simulink model "CSI_0313_SDC"  (R2019b)
settings: Solver=FixedStepDiscrete  StartTime=0.0  StopTime=Tstop  FixedStep=Tdelt  MaxStep=1e-4  RelTol=1e-3
values from neighbouring files (symbols this model uses):
  C = 12e-6    (= 1.2e-05)    [Inputparameter.m]
  Cdc = 4.76*10^-3    (= 0.00476)    [Inputparameter.m]
  Cemc = 1.5e-6    (= 1.5e-06)    [Inputparameter.m]
  enb = 0    [Run.m]
  fanalog = 7000    [Run.m]
  fTs = Update/18000    (= 0.000111111111111)    [Run.m]
  Ibase = 43*sqrt(2)    [Inputparameter.m]
  K120 = 0.0    (= 0)    [Run.m]
  K21 = 0.0    (= 0)    [Run.m]
  K5 = 0.0    (= 0)    [Run.m]
  K7 = 0.0    (= 0)    [Run.m]
  Kipll = 1.0    (= 1)    [Run.m]
  Klim = 1.03    [Run.m]
  Kpll = 20.0    (= 20)    [Run.m]
  Kpr = 0.9*Ibase/(Vbase)    [Run.m]
  Lgrid = 7.717e-4*10    (= 0.007717)    [Run.m]
  Lline = 60e-6    (= 6e-05)    [Inputparameter.m]
  Lpwm = 184.8e-6    (= 0.0001848)    [Inputparameter.m]
  mode = 1    [Run.m]
  Nsw = 18000/fbase    [Run.m]
  Qbpf = 1.0    (= 1)    [Run.m]
  Qpr = 1.0    (= 1)    [Run.m]
  Qs = 1    [Run.m]
  Rc = 10e-3    (= 0.01)    [Inputparameter.m]
  Remc = 1e-3    (= 0.001)    [Inputparameter.m]
  Rgrid = 2*pi*fbase*Lgrid/XR    [Run.m]
  Rline = 4.95e-3    (= 0.00495)    [Inputparameter.m]
  Rpre = 2.2    [Inputparameter.m]
  Rpwm = 6.2e-3    (= 0.0062)    [Inputparameter.m]
  Tdelt = (fTs)/(200*Update)    (= 2.77777777778e-07)    [Run.m]
  Tdt = 1.27e-6    (= 1.27e-06)    [Run.m]
  tstart = 0.2    [Run.m]
  Update = 2    [Run.m]
  Vbase = 400*sqrt(2/3)    [Inputparameter.m]
undefined symbols (not defined in the file or in its folder): sigbuilder_block
libraries: powerlib x54
(part 1 of 4)
settings Model: SimulationMode=accelerator  Creator=seyuoka  LastModifiedBy=INANPAN1
settings DataIOCC: ReturnWorkspaceOutputs=off
settings OptimizationCC: EfficientMapNaN2IntZero=off
settings DebuggingCC: ArithmeticOperatorsInVariantConditions=warning
settings HardwareCC: TargetBitPerPointer=64  TargetBitPerSizeT=64  TargetBitPerPtrDiffT=64  TargetLongLongMode=on  TargetIntDivRoundTo=Zero  TargetEndianess=LittleEndian  TargetWordSize=64  TargetHWDeviceType=MATLAB Host  ProdEqTarget=off
settings SFSimCC: SimUseLocalCustomCode=off  CustomCodeUndefinedFunction=UseInterfaceOnly
settings RTWCC: RTWUseLocalCustomCode=off
settings CodeAppCC: MaxIdLength=128
settings GRTTargetCC: TargetLangStandard=C89/C90 (ANSI)  CombineOutputUpdateFcns=off  GRTInterface=on
settings SimscapeCC: SimscapeNormalizeSystem=off

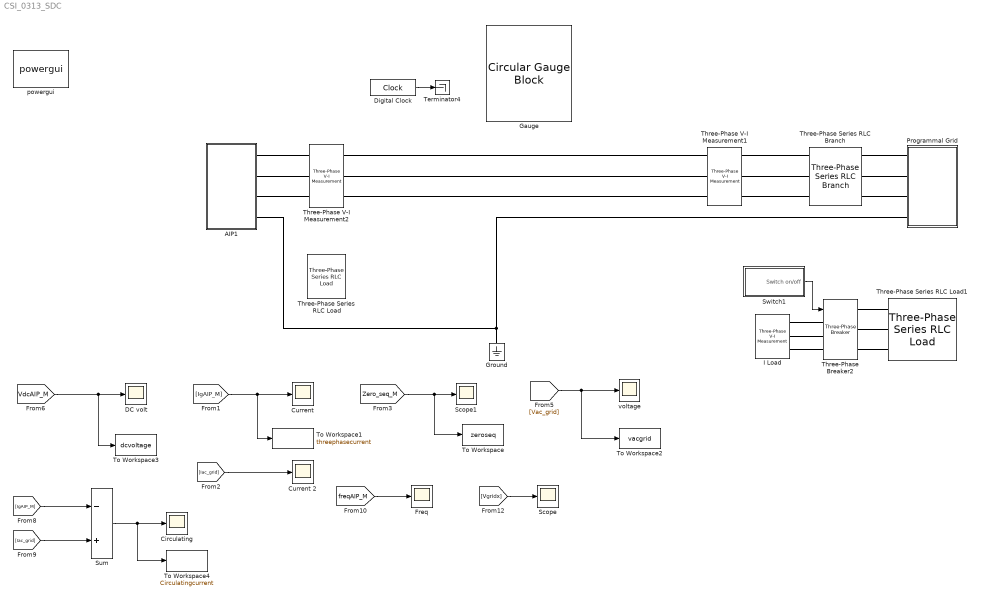
== system CSI_0313_SDC ==
  AIP1 : Subsystem
  Circulating : Scope
  "Current " : Scope
  Current 2 : Scope
  DC volt : Scope
  Digital Clock : DigitalClock  SampleTime=0.001
  Freq : Scope
  Gauge : CircularGaugeBlock  ScaleMax=1  TickInterval=0.1
  Ground : powerlib/Elements/Ground  LConnTagsString=a
      settings: SourceProductName=Simscape Electrical
  I Load : powerlib/Measurements/Three-Phase V-I Measurement  VoltageMeasurement=phase-to-ground  SetLabelV=on  LabelV=VLoad  Vpu=off  VpuLL=off  CurrentMeasurement=yes  SetLabelI=on  LabelI=ILoad  Ipu=off  Pbase=100e6  Vbase=500e3  OutputType=Complex  PhasorSimulation=off  PSBequivalent=0
      settings: SourceProductName=Simscape Electrical
  Programmal Grid : Subsystem  AncestorBlock=AIP_Library0107/Programmal Grid
  Scope : Scope
  Scope1 : Scope
  Sum : Sum  Inputs=-+
  Switch1 : Subsystem  Tag=STV Subsys  LoadFcn=sigbuilder_block('load');  StartFcn=sigbuilder_block('start');  StopFcn=sigbuilder_block('stop');  ClipboardFcn=sigbuilder_block('clipboard');  mask(Sigbuilder block){tuvar=[0:10]}
      mask help: Simulink:masks:SigbuilderBlock_MD
      mask init:
      | if ~strcmp(get_param(bdroot(gcbh),'SimulationStatus'),'stopped') tuvar = sigbuilder_block('maskInit'); end
      settings: CopyFcn=sigbuilder_block('copy');  DeleteFcn=sigbuilder_block('delete');  ModelCloseFcn=sigbuilder_block('modelClose');  PreSaveFcn=sigbuilder_block('preSave');  PauseFcn=sigbuilder_block('pause');  ContinueFcn=sigbuilder_block('continue');  NameChangeFcn=sigbuilder_block('namechange');  OpenFcn=sigbuilder_block('open',[467 144 551 302 ]);  CloseFcn=sigbuilder_block('close');
      mask Display: plot(0, 0, 100, 100,[2, 2, 32, 32, 2], [68, 8, 8, 68, 68],[32, 2], [38, 38], [32, 19, 2],[53, 60, 44], [32, 17, 17, 2],[16, 16, 31, 31]);txt = getActiveGroup(gcbh);text(2, 100, txt,'verticalAlignment', 'top');
  Terminator4 : Terminator
  Three-Phase Series RLC Branch : powerlib/Elements/Three-Phase Series RLC Branch  LConnTagsString=A|B|C  RConnTagsString=A|B|C  BranchType=RL  Resistance=Rgrid  Inductance=Lgrid  Capacitance=1e-6  Measurements=None
      settings: SourceProductName=Simscape Electrical
  Three-Phase Series RLC Load : powerlib/Elements/Three-Phase Series RLC Load  LConnTagsString=A|B|C  Configuration=Y (floating)  NominalVoltage=400  Vabc=[1e3 1e3 1e3]  Vabcp=[1e3 1e3 1e3]  NominalFrequency=50  UnbalancedPower=off  ActivePower=5000  InductivePower=0  CapacitivePower=0  Pabc=[10e3 9e3 11e3]  QLabc=[100 90 110]  QCabc=[100 90 110]  Pabcp=[10e3 9e3 11e3]  QLabcp=[100 90 110]  QCabcp=[100 90 110]  Measurements=None  LoadType=constant Z
      settings: SourceProductName=Simscape Electrical
  Three-Phase Series RLC Load1 : powerlib/Elements/Three-Phase Series RLC Load  LConnTagsString=A|B|C  Configuration=Y (grounded)  NominalVoltage=400  Vabc=[230 230 230]  Vabcp=[400 400 400]  NominalFrequency=50  UnbalancedPower=off  ActivePower=6e3  InductivePower=20e3  CapacitivePower=0  Pabc=[1 3e3 1]  QLabc=[0 16e3 0]  QCabc=[0 0 0]  Pabcp=[1 3e3 1]  QLabcp=[0 6e3 0]  QCabcp=[0 0 0]  Measurements=None  LoadType=constant Z
      settings: SourceProductName=Simscape Electrical
  Three-Phase V-I Measurement1 : powerlib/Measurements/Three-Phase V-I Measurement  VoltageMeasurement=phase-to-ground  SetLabelV=on  LabelV=Vac_grid  Vpu=off  VpuLL=off  CurrentMeasurement=yes  SetLabelI=on  LabelI=Iac_grid  Ipu=off  Pbase=100e6  Vbase=500e3  OutputType=Complex  PhasorSimulation=off  PSBequivalent=0
      settings: SourceProductName=Simscape Electrical
  Three-Phase V-I Measurement2 : powerlib/Measurements/Three-Phase V-I Measurement  VoltageMeasurement=no  SetLabelV=on  LabelV=vacgrid  Vpu=off  VpuLL=off  CurrentMeasurement=yes  SetLabelI=on  LabelI=IgAIP_M  Ipu=off  Pbase=100e6  Vbase=500e3  OutputType=Complex  PhasorSimulation=off  PSBequivalent=0
      settings: SourceProductName=Simscape Electrical
  Three-Phase Breaker2 : powerlib/Elements/Three-Phase Breaker  InitialState=open  SwitchA=on  SwitchB=on  SwitchC=on  SwitchTimes=1.2  External=on  BreakerResistance=0.01  SnubberResistance=1e6  SnubberCapacitance=inf  Measurements=None
      settings: SourceProductName=Simscape Electrical
  To Workspace : ToWorkspace  VariableName=zeroseq  SaveFormat=Timeseries  SampleTime=-1
  To Workspace1 : ToWorkspace  VariableName=threephasecurrent  SaveFormat=Timeseries  SampleTime=-1
  To Workspace2 : ToWorkspace  VariableName=vacgrid  SaveFormat=Timeseries  SampleTime=-1
  To Workspace3 : ToWorkspace  VariableName=dcvoltage  SaveFormat=Timeseries  SampleTime=-1
  To Workspace4 : ToWorkspace  VariableName=Circulatingcurrent  SaveFormat=Timeseries  SampleTime=-1
  powergui : powerlib/powergui  Priority=1  SimulationMode=Discrete  SampleTime=Tdelt  frequency=50  Iterations=50  frequencyindice=0  Pbase=100e6  ErrMax=1e-4  UnitsV=kV  UnitsW=MW  buscounter=0  FunctionMessages=off  echomessages=off  EnableUseOfTLC=off  CurrentSourceSwitches=off  DisableSnubberDevices=off  DisableRonSwitches=off  DisableVfSwitches=off  DisplayEquations=off  AutomaticDiscreteSolvers=off  SolverType=Tustin/Backward Euler (TBE)  Interpol=off  ExternalGateDelay=off  methode=off  Ts=100  x0status=blocks  SPID=off  SwTol=0  HookPort=off  NonlinearTolerance=1e-4  nMaxIteration=100  ContinueOnMaxIteration=off  RestoreLinks=warning  ResistiveCurrentMeasurement=off  Frange=[0:2:500]  Ylog=off  Xlog=on  ShowGrid=off  save=off  variable=ZData  structure=AIPcurrent  ZoomFFT=on  StartTime=0.8  cycles=5  DisplayStyle=1  fundamental=50  FreqAxis=off  MaxFrequency=5000  frequencyindicesteady=1  RmsSteady=1  display=off
      settings: SourceProductName=Simscape Electrical
  voltage : Scope
  wires:
  Digital Clock/1 -> Terminator4/1
  [Vac_grid] -> voltage/1, To Workspace2/1
  [IgAIP_M] -> Sum/1
  [Iac_grid] -> Sum/2
  Sum/1 -> To Workspace4/1, Circulating/1
  [freqAIP_M] -> Freq/1
  [Vgridx] -> Scope/1
  [VdcAIP_M] -> To Workspace3/1, DC volt/1
  [IgAIP_M] -> To Workspace1/1, "Current "/1
  [Zero_seq_M] -> Scope1/1, To Workspace/1
  [Iac_grid] -> Current 2/1
  Switch1/1(Switch on/off) -> Three-Phase Breaker2/1
  connections:
  Three-Phase V-I Measurement2/RConn1 -- Three-Phase V-I Measurement1/LConn1
  Three-Phase V-I Measurement1/LConn3 -- Three-Phase V-I Measurement2/RConn3
  Three-Phase V-I Measurement2/RConn2 -- Three-Phase V-I Measurement1/LConn2
  Three-Phase V-I Measurement1/RConn1 -- Three-Phase Series RLC Branch/LConn1
  Three-Phase V-I Measurement1/RConn2 -- Three-Phase Series RLC Branch/LConn2
  Three-Phase V-I Measurement1/RConn3 -- Three-Phase Series RLC Branch/LConn3
  Programmal Grid/RConn4 -- AIP1/RConn4 -- Ground/LConn1
  Three-Phase Series RLC Branch/RConn3 -- Programmal Grid/RConn3
  Three-Phase Series RLC Branch/RConn2 -- Programmal Grid/RConn2
  Three-Phase Series RLC Branch/RConn1 -- Programmal Grid/RConn1
  Three-Phase V-I Measurement2/LConn1 -- AIP1/RConn1
  Three-Phase V-I Measurement2/LConn2 -- AIP1/RConn2
  Three-Phase V-I Measurement2/LConn3 -- AIP1/RConn3
  Three-Phase Series RLC Load1/LConn3 -- Three-Phase Breaker2/RConn3
  I Load/RConn1 -- Three-Phase Breaker2/LConn1
  I Load/RConn2 -- Three-Phase Breaker2/LConn2
  Three-Phase Series RLC Load1/LConn2 -- Three-Phase Breaker2/RConn2
  I Load/RConn3 -- Three-Phase Breaker2/LConn3
  Three-Phase Series RLC Load1/LConn1 -- Three-Phase Breaker2/RConn1

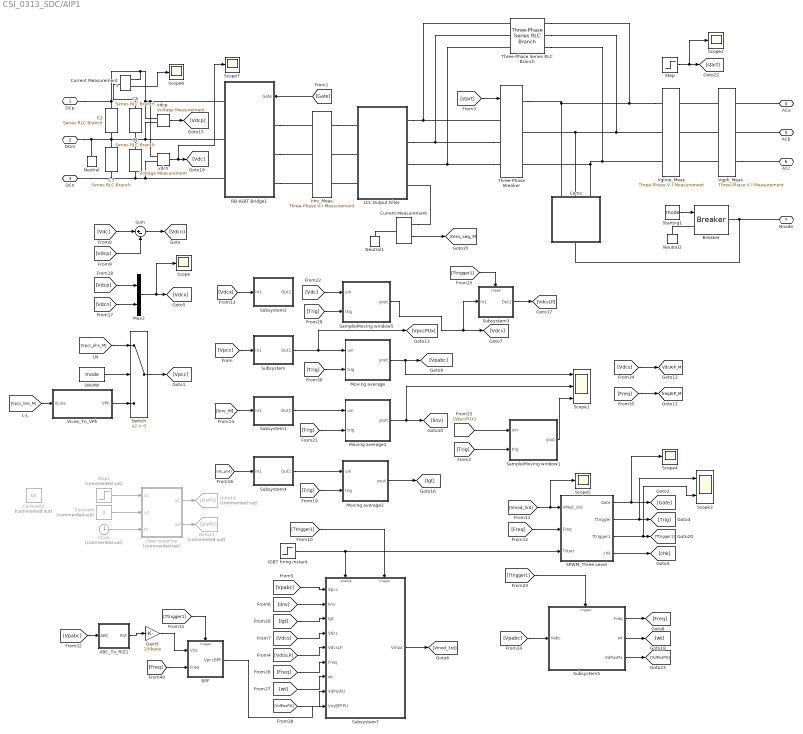
== system CSI_0313_SDC/AIP1 ==
  3W/4W : Constant  Value=mode
  ABC_To_RIZ1 : MATLAB Function  TreatAsAtomicUnit=on
  "BPF " : Subsystem
  Breaker : powerlib/Elements/Breaker  InitialState=0  SwitchingTimes="[1/60  5/60]"  External=on  BreakerResistance=1e-6  SnubberResistance=1e6  SnubberCapacitance=inf  Measurements=None  MoreParameters=on  NoBreakLoop=off
      settings: SourceProductName=Simscape Electrical
  C1 : powerlib/Elements/Series RLC Branch  LConnTagsString=__new0  RConnTagsString=__new0  BranchType=C  Resistance=Rc  Inductance=Lpwm  SetiL0=off  InitialCurrent=0  Capacitance=Cdc  Setx0=on  InitialVoltage=320  Measurements=None
      settings: SourceProductName=Simscape Electrical
  C2 : powerlib/Elements/Series RLC Branch  LConnTagsString=__new0  RConnTagsString=__new0  BranchType=R  Resistance=120e3  Inductance=Lpwm  SetiL0=off  InitialCurrent=0  Capacitance=Cdc  Setx0=on  InitialVoltage=300  Measurements=None
      settings: SourceProductName=Simscape Electrical
  C3 : powerlib/Elements/Series RLC Branch  LConnTagsString=__new0  RConnTagsString=__new0  BranchType=R  Resistance=120e3  Inductance=Lpwm  SetiL0=off  InitialCurrent=0  Capacitance=Cdc  Setx0=on  InitialVoltage=300  Measurements=None
      settings: SourceProductName=Simscape Electrical
  C8 : powerlib/Elements/Series RLC Branch  LConnTagsString=__new0  RConnTagsString=__new0  BranchType=C  Resistance=Rc  Inductance=Lpwm  SetiL0=off  InitialCurrent=0  Capacitance=Cdc  Setx0=on  InitialVoltage=320  Measurements=None
      settings: SourceProductName=Simscape Electrical
  Cemc : Subsystem
  Clock : Clock  Commented=on
  Constant : Constant  Commented=on  Value=0
  Constant2 : Constant  Commented=on  Value=Qs
  Current Measurement : powerlib/Measurements/Current Measurement  PhasorSimulation=off  OutputType=Complex  PSBequivalent=0
      settings: SourceProductName=Simscape Electrical
  Current Measurement1 : powerlib/Measurements/Current Measurement  PhasorSimulation=off  OutputType=Complex  PSBequivalent=0
      settings: SourceProductName=Simscape Electrical
  Gain5 : Gain  Gain=1/Vbase
  Goto14 : Goto  Commented=on  GotoTag=PrefPU
  Goto21 : Goto  Commented=on  GotoTag=QrefPU
  IGBT firing instant : Step  Time=0.11  SampleTime=0
  Iinv_Meas : powerlib/Measurements/Three-Phase V-I Measurement  VoltageMeasurement=no  SetLabelV=off  LabelV=Vabc  Vpu=off  VpuLL=off  CurrentMeasurement=yes  SetLabelI=on  LabelI=Iinv_M  Ipu=off  Pbase=100e6  Vbase=500e3  OutputType=Complex  PhasorSimulation=off  PSBequivalent=0
      settings: SourceProductName=Simscape Electrical
  LCL Output Filter : Subsystem  AncestorBlock=AIP_Library0107/LCL Output Filter
  Moving average : MATLAB Function  Priority=-1  AncestorBlock=AIP_Library0123/Sample//Moving window  TreatAsAtomicUnit=on  mask{iNumAvg=4, iNumDly=1, ubase=1}
      mask prompts: iNumAvg "Sample points"; iNumDly "Delay points"; ubase "Base Value"
  Moving average1 : MATLAB Function  Priority=-1  AncestorBlock=AIP_Library0123/Sample//Moving window  TreatAsAtomicUnit=on  mask{iNumAvg=4, iNumDly=1, ubase=1}
      mask prompts: iNumAvg "Sample points"; iNumDly "Delay points"; ubase "Base Value"
  Moving average2 : MATLAB Function  Priority=-1  AncestorBlock=AIP_Library0123/Sample//Moving window  TreatAsAtomicUnit=on  mask{iNumAvg=4, iNumDly=1, ubase=1}
      mask prompts: iNumAvg "Sample points"; iNumDly "Delay points"; ubase "Base Value"
  Mux2 : Mux  Inputs=2
  Neutral : powerlib/Elements/Neutral  LConnTagsString=a  NodeNumber=10
      settings: SourceProductName=Simscape Electrical  SourceProductBaseCode=PS
  Neutral1 : powerlib/Elements/Neutral  LConnTagsString=a  NodeNumber=10
      settings: SourceProductName=Simscape Electrical  SourceProductBaseCode=PS
  Neutral2 : powerlib/Elements/Neutral  LConnTagsString=a  NodeNumber=10
      settings: SourceProductName=Simscape Electrical  SourceProductBaseCode=PS
  RB-IGBT Bridge1 : Subsystem  AncestorBlock=AIP_Library0107/RB-IGBT Bridge
  SPWM_Three Level : Subsystem  mask{ID=1, Tdelt=Tdelt, Tdt=Tdt}
      mask prompts: ID "Unit Serial Number"; Tdelt "Simulation Step [s]"; Tdt "Dead time [s]"
  Sample/Moving window1 : MATLAB Function  Priority=-1  AncestorBlock=AIP_Library0123/Sample//Moving window  TreatAsAtomicUnit=on  mask{iNumAvg=1, iNumDly=1, ubase=Vbase}
      mask prompts: iNumAvg "Sample points"; iNumDly "Delay points"; ubase "Base Value"
  Sample/Moving window5 : MATLAB Function  Priority=-1  AncestorBlock=AIP_Library0123/Sample//Moving window  TreatAsAtomicUnit=on  mask{iNumAvg=1, iNumDly=1, ubase=1}
      mask prompts: iNumAvg "Sample points"; iNumDly "Delay points"; ubase "Base Value"
  Scope{,2,4..7} (6 alike) : Scope
  Scope1 : Scope  NumInputPorts=3
  Scope3 : Scope  NumInputPorts=2
  Startsig1 : Constant  Value=mode
  Step : Step  Time=0.1  SampleTime=0
  Step response : MATLAB Function  Commented=on  TreatAsAtomicUnit=on  mask{enb=enb}
      mask prompts: enb "enable"
  Step1 : Step  Commented=on  Time=0.2  After=0.5  SampleTime=0
  Subsystem : Subsystem
  Subsystem1 : Subsystem
  Subsystem2 : Subsystem
  Subsystem3 : Subsystem
  Subsystem4 : Subsystem
  Subsystem5 : Subsystem
  Subsystem7 : Subsystem
  Sum : Sum  Inputs=|+-
  Switch : Switch  Criteria=u2 > Threshold
  Three-Phase Series RLC Branch : powerlib/Elements/Three-Phase Series RLC Branch  LConnTagsString=A|B|C  RConnTagsString=A|B|C  BranchType=R  Resistance=Rpre  Inductance=1e-3  Capacitance=1e-6  Measurements=None
      settings: SourceProductName=Simscape Electrical
  Three-Phase Breaker : powerlib/Elements/Three-Phase Breaker  InitialState=open  SwitchA=on  SwitchB=on  SwitchC=on  SwitchTimes=tstart  External=on  BreakerResistance=1e-6  SnubberResistance=1e6  SnubberCapacitance=inf  Measurements=None
      settings: SourceProductName=Simscape Electrical
  VLine_To_VPh : MATLAB Function  AncestorBlock=AIP_Library0107/VLine_To_VPh  TreatAsAtomicUnit=on
  Vgline_Meas : powerlib/Measurements/Three-Phase V-I Measurement  VoltageMeasurement=phase-to-phase  SetLabelV=on  LabelV=Vpcc_line_M  Vpu=off  VpuLL=off  CurrentMeasurement=no  SetLabelI=off  LabelI=vpccabbc  Ipu=off  Pbase=100e6  Vbase=500e3  OutputType=Complex  PhasorSimulation=off  PSBequivalent=0
      settings: SourceProductName=Simscape Electrical
  Vgph_Meas : powerlib/Measurements/Three-Phase V-I Measurement  VoltageMeasurement=phase-to-ground  SetLabelV=on  LabelV=Vpcc_phn_M  Vpu=off  VpuLL=off  CurrentMeasurement=no  SetLabelI=off  LabelI=vpccabbc  Ipu=off  Pbase=100e6  Vbase=500e3  OutputType=Complex  PhasorSimulation=off  PSBequivalent=0
      settings: SourceProductName=Simscape Electrical
  vdcn : powerlib/Measurements/Voltage Measurement  PhasorSimulation=off  OutputType=Magnitude  PSBequivalent=0
      settings: SourceProductName=Simscape Electrical
  vdcp : powerlib/Measurements/Voltage Measurement  PhasorSimulation=off  OutputType=Magnitude  PSBequivalent=0
      settings: SourceProductName=Simscape Electrical
  DCp : PMIOPort  Side=Left
  DCm : PMIOPort  Port=2  Side=Left
  DCn : PMIOPort  Port=3  Side=Left
  ACa : PMIOPort  Port=4  Side=Right
  ACb : PMIOPort  Port=5  Side=Right
  ACc : PMIOPort  Port=6  Side=Right
  Nnode : PMIOPort  Port=7  Side=Right
  tag scope: VdcAIP_M=global, Zero_seq_M=global, freqAIP_M=global
  wires:
  [Vpcc_line_M] -> VLine_To_VPh/1(VLine)
  SPWM_Three Level/2(Ttrigger) -> Scope3/1, [Trig]
  Mux2/1 -> Scope/1, [Vdcx]
  SPWM_Three Level/1(Gate) -> Scope4/1, [Gate]
  SPWM_Three Level/3(Ttrigger1) -> Scope3/2, [Ttrigger1]
  SPWM_Three Level/4(chk) -> [chk]
  Clock/1 -> Step response/3(tx)
  VLine_To_VPh/1(VPh) -> Switch/3
  3W/4W/1 -> Switch/2
  [Vpcc_phn_M] -> Switch/1
  [Vdcp] -> Mux2/1
  [Vdcn] -> Mux2/2
  Switch/1 -> [Vpcc]
  Step response/1(y1) -> Goto14/1
  Step response/2(y2) -> Goto21/1
  [Vpabc] -> Subsystem7/1(Vpcc)
  [Iinv] -> Subsystem7/2(Iinv)
  [Vdcs] -> Subsystem7/4(Vdcs)
  [Ttrigger1] -> Subsystem7/Trigger
  Subsystem7/1(Vmod) -> [Vmod_3rd]
  Subsystem5/1(Freq) -> [Freq]
  [Vmod_3rd] -> SPWM_Three Level/1(VMod_3rd), Scope5/1
  [Freq] -> SPWM_Three Level/2(Freq)
  [Vdcs] -> [VdcAIP_M]
  [Freq] -> [freqAIP_M]
  Current Measurement/1 -> [Zero_seq_M]
  vdcn/1 -> Scope7/1, [Vdc]
  [Gate] -> RB-IGBT Bridge1/1(Gate)
  Step/1 -> Scope2/1, [start]
  Startsig1/1 -> Breaker/1
  vdcp/1 -> [Vdcp]
  [Trig] -> Sample/Moving window5/2(trig)
  [Trig] -> Moving average1/2(trig)
  [Vdcx] -> Subsystem2/1(In1)
  [Vpcc] -> Subsystem/1(In1)
  [Trig] -> Moving average/2(trig)
  [Ttrigger1] -> Subsystem3/Trigger
  Subsystem/1(Out1) -> [VpccPUx], Moving average/1(uin)
  [Iinv_M] -> Subsystem1/1(In1)
  Subsystem1/1(Out1) -> Moving average1/1(uin)
  Moving average/1(yout) -> Scope1/1, [Vpabc]
  Moving average1/1(yout) -> Scope1/2, [Iinv]
  [Trig] -> Sample/Moving window1/2(trig)
  Sample/Moving window1/1(yout) -> Scope1/3
  [VpccPUx] -> Sample/Moving window1/1(uin)
  Step1/1 -> Step response/1(u1)
  Constant/1 -> Step response/2(u2)
  Subsystem4/1(Out1) -> Moving average2/1(uin)
  [Iac_grid] -> Subsystem4/1(In1)
  [Trig] -> Moving average2/2(trig)
  Moving average2/1(yout) -> [Igt]
  [Igt] -> Subsystem7/3(Igt)
  [start] -> Three-Phase Breaker/1
  IGBT firing instant/1 -> SPWM_Three Level/3(Tstart), Subsystem7/Enable
  Subsystem3/1(Out1) -> [VdcsLP]
  [VdcsLP] -> Subsystem7/5(VdcsLP)
  [Vdc] -> Sum/1
  [Vdcp] -> Sum/2
  Sum/1 -> [Vdcn]
  [Vdc] -> Sample/Moving window5/1(uin)
  Sample/Moving window5/1(yout) -> Subsystem3/1(In1), [Vdcs]
  [Ttrigger1] -> Subsystem5/Trigger
  [Vpabc] -> Subsystem5/1(Vabc)
  [Freq] -> Subsystem7/6("Freq ")
  Subsystem5/2(wt) -> [wt]
  Subsystem5/3(VdPosPU) -> [VdPosPU]
  [wt] -> Subsystem7/7(wt)
  [VdPosPU] -> Subsystem7/8(VdPosPU)
  Current Measurement1/1 -> Scope6/1
  "BPF "/1(VpccBPF) -> Subsystem7/9(VrizBPFPU)
  [Freq] -> "BPF "/2(Freq)
  Gain5/1 -> "BPF "/1(Vriz)
  [Ttrigger1] -> "BPF "/Trigger
  [Vpabc] -> ABC_To_RIZ1/1(ABC)
  ABC_To_RIZ1/1(RIZ) -> Gain5/1
  connections:
  vdcp/LConn1 -- Current Measurement1/RConn1 -- C2/LConn1 -- DCp/RConn1 -- vdcn/LConn1 -- RB-IGBT Bridge1/RConn1
  Vgline_Meas/LConn1 -- Three-Phase Series RLC Branch/RConn1 -- Three-Phase Breaker/RConn1 -- Cemc/LConn1
  Three-Phase Breaker/RConn3 -- Vgline_Meas/LConn3 -- Three-Phase Series RLC Branch/RConn3 -- Cemc/LConn3
  C8/RConn1 -- C3/LConn1 -- DCm/RConn1 -- Neutral/LConn1 -- C2/RConn1 -- RB-IGBT Bridge1/RConn2 -- vdcp/LConn2 -- C1/LConn1
  Three-Phase Breaker/LConn3 -- LCL Output Filter/RConn3 -- Three-Phase Series RLC Branch/LConn3
  Three-Phase Breaker/RConn2 -- Vgline_Meas/LConn2 -- Three-Phase Series RLC Branch/RConn2 -- Cemc/LConn2
  Three-Phase Breaker/LConn2 -- LCL Output Filter/RConn2 -- Three-Phase Series RLC Branch/LConn2
  Cemc/RConn1 -- Breaker/RConn1 -- Nnode/RConn1
  RB-IGBT Bridge1/RConn3 -- vdcn/LConn2 -- C1/RConn1 -- C3/RConn1 -- DCn/RConn1
  Three-Phase Series RLC Branch/LConn1 -- LCL Output Filter/RConn1 -- Three-Phase Breaker/LConn1
  Current Measurement/LConn1 -- Neutral1/LConn1
  ACa/RConn1 -- Vgph_Meas/RConn1
  RB-IGBT Bridge1/LConn2 -- Iinv_Meas/LConn2
  Neutral2/LConn1 -- Breaker/LConn1
  RB-IGBT Bridge1/LConn3 -- Iinv_Meas/LConn3
  Vgph_Meas/RConn3 -- ACc/RConn1
  Vgph_Meas/LConn2 -- Vgline_Meas/RConn2
  ACb/RConn1 -- Vgph_Meas/RConn2
  RB-IGBT Bridge1/LConn1 -- Iinv_Meas/LConn1
  Iinv_Meas/RConn1 -- LCL Output Filter/LConn1
  LCL Output Filter/LConn2 -- Iinv_Meas/RConn2
  Vgph_Meas/LConn1 -- Vgline_Meas/RConn1
  Vgph_Meas/LConn3 -- Vgline_Meas/RConn3
  LCL Output Filter/LConn3 -- Iinv_Meas/RConn3
  Current Measurement/RConn1 -- LCL Output Filter/RConn4
  Current Measurement1/LConn1 -- C8/LConn1

== system CSI_0313_SDC/Programmal Grid ==
  Clock : Clock
  Phase A : powerlib/Electrical Sources/Controlled Voltage Source  Initialize=on  Source_Type=AC  Amplitude=0  Phase=0  Frequency=0  Measurements=None
      settings: SourceProductName=Simscape Electrical
  Phase B : powerlib/Electrical Sources/Controlled Voltage Source  Initialize=on  Source_Type=AC  Amplitude=0  Phase=0  Frequency=0  Measurements=None
      settings: SourceProductName=Simscape Electrical
  Phase C : powerlib/Electrical Sources/Controlled Voltage Source  Initialize=on  Source_Type=AC  Amplitude=0  Phase=0  Frequency=0  Measurements=None
      settings: SourceProductName=Simscape Electrical
  "Programmal Grid " : MATLAB Function  TreatAsAtomicUnit=on  mask{Tdelt=Tdelt, K5=K5, K7=K7, K21=K21, K120=K120}
      mask prompts: Tdelt "Simulation time step"; K5 "5th component"; K7 "7th component"; K21 "21th component"; K120 "120th component"
  Three-Phase V-I Measurement1 : powerlib/Measurements/Three-Phase V-I Measurement  VoltageMeasurement=phase-to-ground  SetLabelV=on  LabelV=Vgridx  Vpu=off  VpuLL=off  CurrentMeasurement=no  SetLabelI=off  LabelI=vpccabbc  Ipu=off  Pbase=100e6  Vbase=500e3  OutputType=Complex  PhasorSimulation=off  PSBequivalent=0
      settings: SourceProductName=Simscape Electrical
  A : PMIOPort  Tag=PMCPort  Side=Right
  B : PMIOPort  Tag=PMCPort  Port=2  Side=Right
  C : PMIOPort  Tag=PMCPort  Port=3  Side=Right
  GND : PMIOPort  Tag=PMCPort  Port=4  Side=Right
  wires:
  "Programmal Grid "/2(ub) -> Phase B/1
  "Programmal Grid "/1(ua) -> Phase A/1
  "Programmal Grid "/3(uc) -> Phase C/1
  Clock/1 -> "Programmal Grid "/1(t)
  connections:
  Phase A/LConn1 -- Phase B/LConn1 -- Phase C/LConn1 -- GND/RConn1
  B/RConn1 -- Three-Phase V-I Measurement1/RConn2
  A/RConn1 -- Three-Phase V-I Measurement1/RConn1
  C/RConn1 -- Three-Phase V-I Measurement1/RConn3
  Phase C/RConn1 -- Three-Phase V-I Measurement1/LConn3
  Phase B/RConn1 -- Three-Phase V-I Measurement1/LConn2
  Three-Phase V-I Measurement1/LConn1 -- Phase A/RConn1

== system CSI_0313_SDC/Switch1 ==
  Demux : Demux  Tag=STV Demux  Outputs=1
  FromWs : FromWorkspace  Tag=STV FromWs  VariableName=tuvar  SampleTime=0
      SigBuilderData=|
      | common.afterFinalStr = 'Extrapolate'
      | common.sampleTime = 0
      | dataSet(1).timeRange = [0 1]
      | dataSet(1).name = 'On 0.2, Off 0.7'
      | dataSet(2).timeRange = [0 1]
      | dataSet(2).name = 'Switch on'
      | dataSet(3).timeRange = [0 1]
      | dataSet(3).name = 'Switch off'
      | sbobj.Groups(1).Name = 'On 0.2, Off 0.7'
      | sbobj.Groups(1).Signals.Name = 'Switch on/off'
      | sbobj.Groups(1).Signals.XData = [0 0.2 0.2 0.7 0.7 1]
      | sbobj.Groups(1).Signals.YData = [0 0 1 1 0 0]
      | sbobj.Groups(1).TimeRange = [0 1]
      | sbobj.Groups(2).Name = 'Switch on'
      | sbobj.Groups(2).Signals.Name = 'Switch on/off'
      | sbobj.Groups(2).Signals.XData = [0 0.4 0.8 1]
      | sbobj.Groups(2).Signals.YData = [1 1 1 1]
      | sbobj.Groups(2).TimeRange = [0 1]
      | sbobj.Groups(3).Name = 'Switch off'
      | sbobj.Groups(3).Signals.Name = 'Switch on/off'
      | sbobj.Groups(3).Signals.XData = [0 0.4 0.8 1]
      | sbobj.Groups(3).Signals.YData = [0 0 0 0]
      | sbobj.Groups(3).TimeRange = [0 1]
  Switch on/off : Outport  Tag=STV Outport  VectorParamsAs1DForOutWhenUnconnected=off
  wires:
  FromWs/1 -> Demux/1
  Demux/1 -> Switch on/off/1

== system CSI_0313_SDC/AIP1/BPF  ==
  Vriz : Inport
  Freq : Inport  Port=2
  Trigger : TriggerPort  TriggerType=falling  VariantControl=Variant  PortDimensions=1
  Demux1 : Demux  Outputs=3
  IIR_BPF_Re1 : MATLAB Function  TreatAsAtomicUnit=on  mask{fQ=Qbpf, fTs=fTs, iMode=IIR2 used as BPF in SOGI}
      mask prompts: fQ "Quality factor"; fTs "Sample time [s]"; iMode "Modes of 2nd-order transfer function"
  IIR_BPF_Re2 : MATLAB Function  TreatAsAtomicUnit=on  mask{fQ=Qbpf, fTs=fTs, iMode=IIR2 used as BPF in SOGI}
      mask prompts: fQ "Quality factor"; fTs "Sample time [s]"; iMode "Modes of 2nd-order transfer function"
  IIR_BPF_Re3 : MATLAB Function  TreatAsAtomicUnit=on  mask{fQ=Qbpf, fTs=fTs, iMode=IIR2 used as BPF in SOGI}
      mask prompts: fQ "Quality factor"; fTs "Sample time [s]"; iMode "Modes of 2nd-order transfer function"
  Mux1 : Mux  Inputs=3
  VpccBPF : Outport
  wires:
  Demux1/1 -> IIR_BPF_Re1/1(u)
  Mux1/1 -> VpccBPF/1
  Freq/1 -> IIR_BPF_Re3/2(fn), IIR_BPF_Re2/2(fn), IIR_BPF_Re1/2(fn)
  IIR_BPF_Re2/1(y) -> Mux1/2
  Demux1/2 -> IIR_BPF_Re2/1(u)
  Vriz/1 -> Demux1/1
  IIR_BPF_Re1/1(y) -> Mux1/1
  Demux1/3 -> IIR_BPF_Re3/1(u)
  IIR_BPF_Re3/1(y) -> Mux1/3

== system CSI_0313_SDC/AIP1/Cemc ==
  RLemc1 : powerlib/Elements/Series RLC Branch  LConnTagsString=__new0  RConnTagsString=__new0  BranchType=RC  Resistance=Remc  Inductance=Lpwm  SetiL0=off  InitialCurrent=0  Capacitance=Cemc  Setx0=off  InitialVoltage=326.6  Measurements=None
      settings: SourceProductName=Simscape Electrical
  RLemc2 : powerlib/Elements/Series RLC Branch  LConnTagsString=__new0  RConnTagsString=__new0  BranchType=RC  Resistance=Remc  Inductance=Lpwm  SetiL0=off  InitialCurrent=0  Capacitance=Cemc  Setx0=off  InitialVoltage=326.6  Measurements=None
      settings: SourceProductName=Simscape Electrical
  RLemc3 : powerlib/Elements/Series RLC Branch  LConnTagsString=__new0  RConnTagsString=__new0  BranchType=RC  Resistance=Remc  Inductance=Lpwm  SetiL0=off  InitialCurrent=0  Capacitance=Cemc  Setx0=off  InitialVoltage=326.6  Measurements=None
      settings: SourceProductName=Simscape Electrical
  ConnA : PMIOPort  Side=Left
  ConnB : PMIOPort  Port=2  Side=Left
  ConnC : PMIOPort  Port=3  Side=Left
  Gnd : PMIOPort  Port=4  Side=Right
  connections:
  RLemc1/LConn1 -- ConnA/RConn1
  RLemc3/RConn1 -- Gnd/RConn1 -- RLemc1/RConn1 -- RLemc2/RConn1
  RLemc2/LConn1 -- ConnB/RConn1
  RLemc3/LConn1 -- ConnC/RConn1

== system CSI_0313_SDC/AIP1/LCL Output Filter ==
  RL : powerlib/Elements/Series RLC Branch  LConnTagsString=__new0  RConnTagsString=__new0  BranchType=RL  Resistance=Rpwm  Inductance=Lpwm  SetiL0=off  InitialCurrent=0  Capacitance=1e-6  Setx0=off  InitialVoltage=0  Measurements=None
      settings: SourceProductName=Simscape Electrical
  RL1 : powerlib/Elements/Series RLC Branch  LConnTagsString=__new0  RConnTagsString=__new0  BranchType=RL  Resistance=Rpwm  Inductance=Lpwm  SetiL0=off  InitialCurrent=0  Capacitance=1e-6  Setx0=off  InitialVoltage=0  Measurements=None
      settings: SourceProductName=Simscape Electrical
  RL2 : powerlib/Elements/Series RLC Branch  LConnTagsString=__new0  RConnTagsString=__new0  BranchType=RL  Resistance=Rpwm  Inductance=Lpwm  SetiL0=off  InitialCurrent=0  Capacitance=1e-6  Setx0=off  InitialVoltage=0  Measurements=None
      settings: SourceProductName=Simscape Electrical
  RL3 : powerlib/Elements/Series RLC Branch  LConnTagsString=__new0  RConnTagsString=__new0  BranchType=RL  Resistance=Rline  Inductance=Lline  SetiL0=off  InitialCurrent=0  Capacitance=1e-6  Setx0=off  InitialVoltage=0  Measurements=None
      settings: SourceProductName=Simscape Electrical
  RL4 : powerlib/Elements/Series RLC Branch  LConnTagsString=__new0  RConnTagsString=__new0  BranchType=RL  Resistance=Rline  Inductance=Lline  SetiL0=off  InitialCurrent=0  Capacitance=1e-6  Setx0=off  InitialVoltage=0  Measurements=None
      settings: SourceProductName=Simscape Electrical
  RL5 : powerlib/Elements/Series RLC Branch  LConnTagsString=__new0  RConnTagsString=__new0  BranchType=RL  Resistance=Rline  Inductance=Lline  SetiL0=off  InitialCurrent=0  Capacitance=1e-6  Setx0=off  InitialVoltage=0  Measurements=None
      settings: SourceProductName=Simscape Electrical
  RL6 : powerlib/Elements/Series RLC Branch  LConnTagsString=__new0  RConnTagsString=__new0  BranchType=RC  Resistance=Rc  Inductance=Lpwm  SetiL0=off  InitialCurrent=0  Capacitance=C  Setx0=off  InitialVoltage=326.6  Measurements=None
      settings: SourceProductName=Simscape Electrical
  RL7 : powerlib/Elements/Series RLC Branch  LConnTagsString=__new0  RConnTagsString=__new0  BranchType=RC  Resistance=Rc  Inductance=Lpwm  SetiL0=off  InitialCurrent=0  Capacitance=C  Setx0=off  InitialVoltage=326.6  Measurements=None
      settings: SourceProductName=Simscape Electrical
  RL8 : powerlib/Elements/Series RLC Branch  LConnTagsString=__new0  RConnTagsString=__new0  BranchType=RC  Resistance=Rc  Inductance=Lpwm  SetiL0=off  InitialCurrent=0  Capacitance=C  Setx0=off  InitialVoltage=326.6  Measurements=None
      settings: SourceProductName=Simscape Electrical
  ConnA : PMIOPort  Side=Left
  Conna : PMIOPort  Port=2  Side=Right
  ConnB : PMIOPort  Port=3  Side=Left
  Connb : PMIOPort  Port=4  Side=Right
  ConnC : PMIOPort  Port=5  Side=Left
  Connc : PMIOPort  Port=6  Side=Right
  "Neutral " : PMIOPort  Port=7  Side=Right
  connections:
  RL4/LConn1 -- RL7/LConn1 -- RL1/RConn1
  RL/LConn1 -- ConnA/RConn1
  RL3/LConn1 -- RL6/LConn1 -- RL/RConn1
  RL5/LConn1 -- RL8/LConn1 -- RL2/RConn1
  RL4/RConn1 -- Connb/RConn1
  RL6/RConn1 -- RL7/RConn1 -- "Neutral "/RConn1 -- RL8/RConn1
  RL1/LConn1 -- ConnB/RConn1
  RL3/RConn1 -- Conna/RConn1
  RL2/LConn1 -- ConnC/RConn1
  RL5/RConn1 -- Connc/RConn1

== system CSI_0313_SDC/AIP1/RB-IGBT Bridge1 ==
  Gate : Inport
  Demux : Demux
  Demux1 : Demux
  Demux2 : Demux
  Demux3 : Demux  Outputs=3
  IGBT/Diode{1..5,12} (6 alike) : powerlib/Power Electronics/IGBT//Diode  Ron=Ron1  Rs=1e6  Cs=Cout  Measurements=off
      settings: SourceProductName=Simscape Electrical
  IGBT/Diode{6..11} (6 alike) : powerlib/Power Electronics/IGBT//Diode  Ron=Ron2  Rs=1e6  Cs=Cout  Measurements=off
      settings: SourceProductName=Simscape Electrical
  positive : PMIOPort  Tag=PMCPort  Side=Right
  netural : PMIOPort  Tag=PMCPort  Port=2  Side=Right
  negative : PMIOPort  Tag=PMCPort  Port=3  Side=Right
  A : PMIOPort  Tag=PMCPort  Port=4  Side=Left
  B : PMIOPort  Tag=PMCPort  Port=5  Side=Left
  C : PMIOPort  Tag=PMCPort  Port=6  Side=Left
  wires:
  Demux3/3 -> Demux2/1  "PulseC"
  Demux3/2 -> Demux1/1  "PulseB"
  Demux3/1 -> Demux/1  "PulseA"
  [PulseC_2n] -> IGBT/Diode4/1
  Demux2/4 -> [PulseC_2n]
  Demux2/3 -> [PulseC_1n]
  Demux2/2 -> [PulseC_2p]
  Demux2/1 -> [PulseC_1p]
  [PulseB_2n] -> IGBT/Diode3/1
  Demux1/4 -> [PulseB_2n]
  Demux1/3 -> [PulseB_1n]
  [PulseB_2p] -> IGBT/Diode8/1
  Demux1/2 -> [PulseB_2p]
  [PulseB_1p] -> IGBT/Diode1/1
  Demux1/1 -> [PulseB_1p]
  [PulseA_2n] -> IGBT/Diode12/1
  Demux/4 -> [PulseA_2n]
  Demux/3 -> [PulseA_1n]
  [PulseA_2p] -> IGBT/Diode6/1
  Demux/2 -> [PulseA_2p]
  [PulseA_1p] -> IGBT/Diode5/1
  Demux/1 -> [PulseA_1p]
  Gate/1 -> Demux3/1
  [PulseA_1n] -> IGBT/Diode7/1
  [PulseB_1n] -> IGBT/Diode9/1
  [PulseC_2p] -> IGBT/Diode10/1
  [PulseC_1n] -> IGBT/Diode11/1
  [PulseC_1p] -> IGBT/Diode2/1
  connections:
  C/RConn1 -- IGBT/Diode4/LConn1 -- IGBT/Diode2/RConn1 -- IGBT/Diode11/LConn1
  netural/RConn1 -- IGBT/Diode10/LConn1 -- IGBT/Diode8/LConn1 -- IGBT/Diode6/LConn1
  A/RConn1 -- IGBT/Diode12/LConn1 -- IGBT/Diode5/RConn1 -- IGBT/Diode7/LConn1
  B/RConn1 -- IGBT/Diode3/LConn1 -- IGBT/Diode1/RConn1 -- IGBT/Diode9/LConn1
  IGBT/Diode2/LConn1 -- positive/RConn1 -- IGBT/Diode1/LConn1 -- IGBT/Diode5/LConn1
  IGBT/Diode4/RConn1 -- negative/RConn1 -- IGBT/Diode12/RConn1 -- IGBT/Diode3/RConn1
  IGBT/Diode7/RConn1 -- IGBT/Diode6/RConn1
  IGBT/Diode9/RConn1 -- IGBT/Diode8/RConn1
  IGBT/Diode11/RConn1 -- IGBT/Diode10/RConn1

== system CSI_0313_SDC/AIP1/SPWM_Three Level ==
  VMod_3rd : Inport
  Freq : Inport  Port=2
  Tstart : Inport  Port=3
  Carrier Gen : MATLAB Function  TreatAsAtomicUnit=on  mask{fdelt=Tdelt}
      mask prompts: fdelt "Simulation Step [s]"
  Constant1 : Constant  Value=Nsw
  Constant2 : Constant  Value=18000
  Constant3 : Constant  Value=55e-6
  Constant4 : Constant  Value=Update
  Constant6 : Constant  Value=Update
  Delay1 : Delay  DelayLength=1  SampleTime=fTs
  Demux1 : Demux  Outputs=3
  Mux : Mux
  Product1 : Product
  Product2 : Product
  Pulse Modulation : MATLAB Function  TreatAsAtomicUnit=on
  Scope1 : Scope
  Scope2 : Scope  NumInputPorts=5
  Step : Step  Time=tstart  Before=-1  SampleTime=0
  Switch : Switch  Criteria=u2 > Threshold
  Tdt Insert : MATLAB Function  TreatAsAtomicUnit=on  mask{tdt=Tdt, fdelt=Tdelt}
      mask prompts: tdt "Dead Time [s]"; fdelt "Simulation step [s]"
  Voltage update timing generator : MATLAB Function  TreatAsAtomicUnit=on
  Voltage update timing generator1 : MATLAB Function  TreatAsAtomicUnit=on
  Gate : Outport
  Ttrigger : Outport  Port=2
  Ttrigger1 : Outport  Port=3
  chk : Outport  Port=4
  wires:
  Mux/1 -> chk/1
  [chk] -> Mux/4
  [Tupdate] -> Mux/3
  [carrier] -> Mux/1
  Voltage update timing generator/1(Tupdate) -> [Tupdate]
  [Ttrigger] -> Voltage update timing generator/1(Trigger)
  [carrier] -> Pulse Modulation/1(carrier)
  Carrier Gen/1(carrier) -> [carrier]
  Carrier Gen/2(sgn) -> [Ttrigger]
  [Freq] -> Carrier Gen/1(fsw)
  Product2/1 -> Switch/1
  Delay1/1 -> Product2/1
  Constant2/1 -> [Freq], Switch/3
  Constant1/1 -> Product2/2
  Step/1 -> Switch/2
  Freq/1 -> Delay1/1
  [Freq] -> Product1/1
  Product1/1 -> Mux/2
  Constant3/1 -> Product1/2
  Switch/1 -> Scope1/1
  Tstart/1 -> Tdt Insert/2(st)
  [Tupdatex] -> Pulse Modulation/3(update)
  Pulse Modulation/1(Pulse) -> Tdt Insert/1(pulse)
  Constant4/1 -> Voltage update timing generator/2(Update)
  Tdt Insert/1(Gate) -> Gate/1
  Constant6/1 -> Voltage update timing generator1/2(Update)
  [Ttrigger] -> Voltage update timing generator1/1(Trigger)
  [Tupdate] -> Ttrigger1/1
  [Ttrigger] -> Ttrigger/1
  Pulse Modulation/2(chk) -> [chk]
  Voltage update timing generator1/1(Tupdate) -> [Tupdatex]
  [Ttrigger] -> Pulse Modulation/2(sgn)
  VMod_3rd/1 -> [VMod_3rd]
  [VMod_3rd] -> Pulse Modulation/4(mod)
  Pulse Modulation/3(chk1) -> [chk1]
  [Tupdatex] -> Scope2/1
  [Ttrigger] -> Scope2/2
  [VMod_3rd] -> Demux1/1
  Demux1/1 -> Scope2/5
  [chk1] -> Scope2/4
  [Tupdate] -> Scope2/3

== system CSI_0313_SDC/AIP1/Subsystem ==
  In1 : Inport
  Demux2 : Demux  Outputs=3
  IIR_1st1 : MATLAB Function  TreatAsAtomicUnit=on  mask{fc=fanalog, fTs=Tdelt}
      mask prompts: fc "Cut-off frequency [Hz]"; fTs "Sample time [s]"
      mask help: 1st-order Low Pass Filter
  IIR_1st2 : MATLAB Function  TreatAsAtomicUnit=on  mask{fc=fanalog, fTs=Tdelt}
      mask prompts: fc "Cut-off frequency [Hz]"; fTs "Sample time [s]"
      mask help: 1st-order Low Pass Filter
  IIR_1st3 : MATLAB Function  TreatAsAtomicUnit=on  mask{fc=fanalog, fTs=Tdelt}
      mask prompts: fc "Cut-off frequency [Hz]"; fTs "Sample time [s]"
      mask help: 1st-order Low Pass Filter
  Mux1 : Mux  Inputs=3
  Out1 : Outport
  wires:
  IIR_1st2/1(y) -> Mux1/2
  In1/1 -> Demux2/1
  Demux2/1 -> IIR_1st1/1(u)
  Demux2/3 -> IIR_1st3/1(u)
  Demux2/2 -> IIR_1st2/1(u)
  IIR_1st3/1(y) -> Mux1/3
  Mux1/1 -> Out1/1
  IIR_1st1/1(y) -> Mux1/1

== system CSI_0313_SDC/AIP1/Subsystem1 ==
  In1 : Inport
  Demux2 : Demux  Outputs=3
  IIR_1st1 : MATLAB Function  TreatAsAtomicUnit=on  mask{fc=fanalog, fTs=Tdelt}
      mask prompts: fc "Cut-off frequency [Hz]"; fTs "Sample time [s]"
      mask help: 1st-order Low Pass Filter
  IIR_1st2 : MATLAB Function  TreatAsAtomicUnit=on  mask{fc=fanalog, fTs=Tdelt}
      mask prompts: fc "Cut-off frequency [Hz]"; fTs "Sample time [s]"
      mask help: 1st-order Low Pass Filter
  IIR_1st3 : MATLAB Function  TreatAsAtomicUnit=on  mask{fc=fanalog, fTs=Tdelt}
      mask prompts: fc "Cut-off frequency [Hz]"; fTs "Sample time [s]"
      mask help: 1st-order Low Pass Filter
  Mux1 : Mux  Inputs=3
  Out1 : Outport
  wires:
  IIR_1st1/1(y) -> Mux1/1
  Mux1/1 -> Out1/1
  IIR_1st3/1(y) -> Mux1/3
  Demux2/2 -> IIR_1st2/1(u)
  Demux2/3 -> IIR_1st3/1(u)
  Demux2/1 -> IIR_1st1/1(u)
  In1/1 -> Demux2/1
  IIR_1st2/1(y) -> Mux1/2

== system CSI_0313_SDC/AIP1/Subsystem2 ==
  In1 : Inport
  Demux2 : Demux  Outputs=2
  IIR_1st1 : MATLAB Function  TreatAsAtomicUnit=on  mask{fc=7000, fTs=Tdelt}
      mask prompts: fc "Cut-off frequency [Hz]"; fTs "Sample time [s]"
      mask help: 1st-order Low Pass Filter
  IIR_1st2 : MATLAB Function  TreatAsAtomicUnit=on  mask{fc=7000, fTs=Tdelt}
      mask prompts: fc "Cut-off frequency [Hz]"; fTs "Sample time [s]"
      mask help: 1st-order Low Pass Filter
  Mux1 : Mux  Inputs=2
  Out1 : Outport
  wires:
  IIR_1st1/1(y) -> Mux1/1
  Mux1/1 -> Out1/1
  Demux2/2 -> IIR_1st2/1(u)
  Demux2/1 -> IIR_1st1/1(u)
  In1/1 -> Demux2/1
  IIR_1st2/1(y) -> Mux1/2

== system CSI_0313_SDC/AIP1/Subsystem3 ==
  In1 : Inport
  Trigger : TriggerPort  VariantControl=Variant  PortDimensions=1
  IIR_1st1 : MATLAB Function  TreatAsAtomicUnit=on  mask{fc=10, fTs=fTs}
      mask prompts: fc "Cut-off frequency [Hz]"; fTs "Sample time [s]"
      mask help: 1st-order Low Pass Filter
  Out1 : Outport
  wires:
  IIR_1st1/1(y) -> Out1/1
  In1/1 -> IIR_1st1/1(u)

== system CSI_0313_SDC/AIP1/Subsystem4 ==
  In1 : Inport
  Demux2 : Demux  Outputs=3
  IIR_1st1 : MATLAB Function  TreatAsAtomicUnit=on  mask{fc=fanalog, fTs=Tdelt}
      mask prompts: fc "Cut-off frequency [Hz]"; fTs "Sample time [s]"
      mask help: 1st-order Low Pass Filter
  IIR_1st2 : MATLAB Function  TreatAsAtomicUnit=on  mask{fc=fanalog, fTs=Tdelt}
      mask prompts: fc "Cut-off frequency [Hz]"; fTs "Sample time [s]"
      mask help: 1st-order Low Pass Filter
  IIR_1st3 : MATLAB Function  TreatAsAtomicUnit=on  mask{fc=fanalog, fTs=Tdelt}
      mask prompts: fc "Cut-off frequency [Hz]"; fTs "Sample time [s]"
      mask help: 1st-order Low Pass Filter
  Mux1 : Mux  Inputs=3
  Out1 : Outport
  wires:
  IIR_1st2/1(y) -> Mux1/2
  In1/1 -> Demux2/1
  Demux2/1 -> IIR_1st1/1(u)
  Demux2/3 -> IIR_1st3/1(u)
  Demux2/2 -> IIR_1st2/1(u)
  IIR_1st3/1(y) -> Mux1/3
  Mux1/1 -> Out1/1
  IIR_1st1/1(y) -> Mux1/1

== system CSI_0313_SDC/AIP1/Subsystem5 ==
  Vabc : Inport
  Trigger : TriggerPort  TriggerType=falling  VariantControl=Variant  PortDimensions=1
  Gain6 : Gain  Gain=1/Vbase
  PLL : Subsystem  mask{fKPPLL=Kpll, fKIPLL=Kipll, fDltMin=-19, fDltMax=19, fFqBase=50, fTs=fTs}
      mask prompts: fKPPLL "PLL Proportional Gain"; fKIPLL "PLL Integral Coefficient"; fDltMin "fDelta Minimum Limitation [rad/s]"; fDltMax "fDelta Maximum Limitation [rad/s]"; fFqBase "Base Frequency [Hz]"; fTs "Sample Time [s]"
  Freq : Outport  VectorParamsAs1DForOutWhenUnconnected=off
  wt : Outport  Port=2  VectorParamsAs1DForOutWhenUnconnected=off
  VdPosPU : Outport  Port=3  VectorParamsAs1DForOutWhenUnconnected=off
  wires:
  PLL/1(f) -> Freq/1
  PLL/3(VdPos) -> VdPosPU/1
  [VabcPU] -> PLL/1(Vabc)
  Vabc/1 -> Gain6/1
  PLL/2(wt) -> wt/1
  Gain6/1 -> [VabcPU]

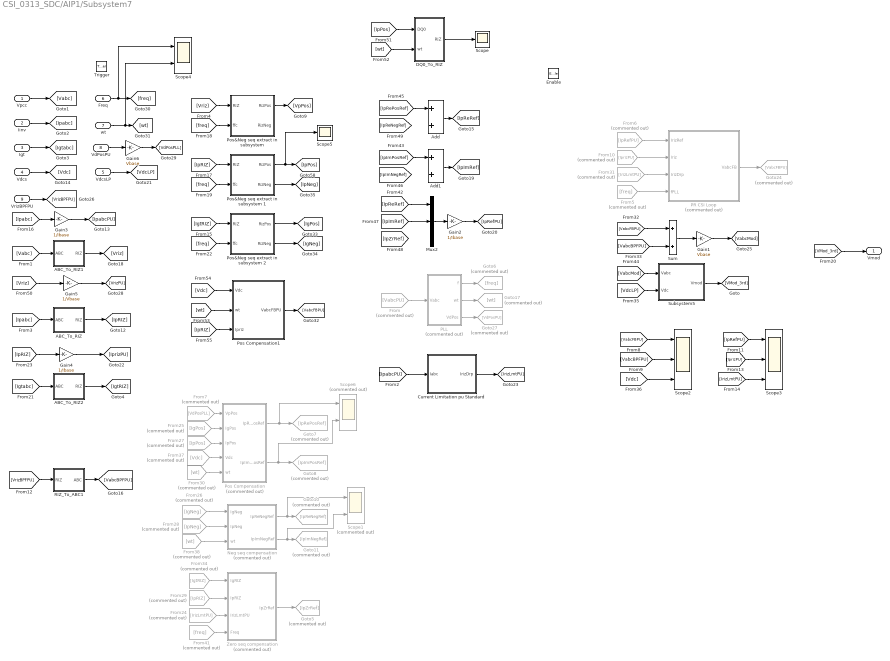
== system CSI_0313_SDC/AIP1/Subsystem7 ==
  Vpcc : Inport
  Iinv : Inport  Port=2
  Igt : Inport  Port=3
  Vdcs : Inport  Port=4
  VdcsLP : Inport  Port=5
  "Freq " : Inport  Port=6
  wt : Inport  Port=7
  VdPosPU : Inport  Port=8
  VrizBPFPU : Inport  Port=9
  Enable : EnablePort
  Trigger : TriggerPort  TriggerType=falling  VariantControl=Variant  PortDimensions=1
  ABC_To_RIZ : MATLAB Function  TreatAsAtomicUnit=on
  ABC_To_RIZ1 : MATLAB Function  TreatAsAtomicUnit=on
  ABC_To_RIZ2 : MATLAB Function  TreatAsAtomicUnit=on
  Add : Sum
  Add1 : Sum
  Current Limitation pu Standard : Subsystem  mask{Klmt=Klim, iRMSNum=180, fTs=fTs}
      mask prompts: Klmt "Limit Ratio"; iRMSNum "RMS Window Points"; fTs "Sample Time [s]"
      mask help: Current Limitation
      mask Display:
      | disp('pu')
      | port_label('input', 1, 'Iabc')
      | port_label('output', 1, 'IrizLmt')
  DQ0_To_RIZ : MATLAB Function  TreatAsAtomicUnit=on  mask{iAxis=orient in A-axis}
      mask prompts: iAxis "Orient Axis Choice"
  From : From  Commented=on  GotoTag=VabcPU
  From10 : From  Commented=on  GotoTag=IprizPU
  From24 : From  Commented=on  GotoTag=IrizLmtPU
  From25 : From  Commented=on  GotoTag=IgPos
  From26 : From  Commented=on  GotoTag=IgNeg
  From27 : From  Commented=on  GotoTag=IpPos
  From28 : From  Commented=on  GotoTag=IpNeg
  From29 : From  Commented=on  GotoTag=IpRIZ
  From30 : From  Commented=on  GotoTag=wt
  From31 : From  Commented=on  GotoTag=IrizLmtPU
  From34 : From  Commented=on  GotoTag=IgtRIZ
  From37 : From  Commented=on  GotoTag=Vdc
  From38 : From  Commented=on  GotoTag=wt
  From41 : From  Commented=on  GotoTag=freq
  From5 : From  Commented=on  GotoTag=freq
  From6 : From  Commented=on  GotoTag=IpRefPU
  From7 : From  Commented=on  GotoTag=VdPosPLL
  Gain1 : Gain  Gain=Vbase
  Gain2 : Gain  Gain=1/Ibase
  Gain3 : Gain  Gain=1/Ibase
  Gain4 : Gain  Gain=1/Ibase
  Gain5 : Gain  Gain=1/Vbase
  Gain6 : Gain  Gain=Vbase
  Goto10 : Goto  Commented=on  GotoTag=IpReNegRef
  Goto11 : Goto  Commented=on  GotoTag=IpImNegRef
  Goto17 : Goto  Commented=on  GotoTag=wt
  Goto24 : Goto  Commented=on  GotoTag=VabcFBPU
  Goto27 : Goto  Commented=on  GotoTag=VdPosPU
  Goto5 : Goto  Commented=on  GotoTag=IpZrRef
  Goto6 : Goto  Commented=on  GotoTag=freq
  Goto7 : Goto  Commented=on  GotoTag=IpRePosRef
  Goto8 : Goto  Commented=on  GotoTag=IpImPosRef
  Mux2 : Mux  Inputs=3
  Neg seq compensation : Subsystem  Commented=on
  PLL : Subsystem  Commented=on  mask{fKPPLL=Kpll, fKIPLL=Kipll, fDltMin=-19, fDltMax=19, fFqBase=50, fTs=fTs}
      mask prompts: fKPPLL "PLL Proportional Gain"; fKIPLL "PLL Integral Coefficient"; fDltMin "fDelta Minimum Limitation [rad/s]"; fDltMax "fDelta Maximum Limitation [rad/s]"; fFqBase "Base Frequency [Hz]"; fTs "Sample Time [s]"
  PR CSI Loop : Subsystem  Commented=on  mask{fKP=Kpr, fKQ=Qpr, fTs=fTs}
      mask prompts: fKP "Proportional Gain"; fKQ "Quality Factor"; fTs "Sample Time [s]"
      mask DialogControl Container5 Prompt: Parameters for PR regulator
      mask Display:
      | disp('PR\n\nCSI Loop')
      | port_label('input', 1, 'IrizRef')
      | port_label('input', 2, 'Iriz')
      | port_label('input', 3, 'IrizLmt')
      | port_label('input', 4, 'ffc')
      | port_label('output', 1, 'VabcFB')
  Pos Compensation : Subsystem  Commented=on
  Pos Compensation1 : Subsystem
  "Pos&Neg seq extract in subsystem " : Subsystem  mask{fQ=1.0, fTs=fTs}
      mask prompts: fQ "Quality Factor"; fTs "Sample Time"
  Pos&Neg seq extract in subsystem 1 : Subsystem  mask{fQ=1.0, fTs=fTs}
      mask prompts: fQ "Quality Factor"; fTs "Sample Time"
  Pos&Neg seq extract in subsystem 2 : Subsystem  mask{fQ=1.0, fTs=fTs}
      mask prompts: fQ "Quality Factor"; fTs "Sample Time"
  RIZ_To_ABC1 : MATLAB Function  TreatAsAtomicUnit=on
  Scope : Scope
  Scope1 : Scope  Commented=on  NumInputPorts=2
  Scope2 : Scope  NumInputPorts=3
  Scope3 : Scope  NumInputPorts=3
  Scope4 : Scope  NumInputPorts=2
  Scope5 : Scope
  Scope6 : Scope  Commented=on  NumInputPorts=2
  Subsystem5 : Subsystem
  Sum : Sum
  Zero seq compensation : Subsystem  Commented=on
  Vmod : Outport
  wires:
  From5/1 -> PR CSI Loop/4(fPLL)
  [VabcFBPU] -> Sum/1
  Subsystem5/1(Vmod) -> [VMod_3rd]
  From10/1 -> PR CSI Loop/2(Iriz)
  Sum/1 -> Gain1/1
  Current Limitation pu Standard/1(IrizDrp) -> [IrizLmtPU]
  Gain1/1 -> [VabcMod]
  PR CSI Loop/1(VabcFB) -> Goto24/1
  [VabcMod] -> Subsystem5/1(Vabc)
  [VMod_3rd] -> Vmod/1
  From6/1 -> PR CSI Loop/1(IrizRef)
  PLL/1(f) -> Goto6/1
  PLL/2(wt) -> Goto17/1
  RIZ_To_ABC1/1(ABC) -> [VabcBPFPU]
  ABC_To_RIZ/1(RIZ) -> [IpRIZ]
  [Ipabc] -> ABC_To_RIZ/1(ABC)
  [Vabc] -> ABC_To_RIZ1/1(ABC)
  From/1 -> PLL/1(Vabc)
  ABC_To_RIZ1/1(RIZ) -> [Vriz]
  PLL/3(VdPos) -> Goto27/1
  [VrizBPFPU] -> RIZ_To_ABC1/1(RIZ)
  Vpcc/1 -> [Vabc]
  Iinv/1 -> [Ipabc]
  [IpabcPU] -> Current Limitation pu Standard/1(Iabc)
  [VabcFBPU] -> Scope2/1
  [VabcBPFPU] -> Scope2/2
  [IpRefPU] -> Scope3/1
  [IprizPU] -> Scope3/2
  [IrizLmtPU] -> Scope3/3
  "Pos&Neg seq extract in subsystem "/1(RizPos) -> [VpPos]
  Pos&Neg seq extract in subsystem 2/1(RizPos) -> [IgPos]
  Pos&Neg seq extract in subsystem 1/2(RizNeg) -> [IpNeg]
  Pos&Neg seq extract in subsystem 2/2(RizNeg) -> [IgNeg]
  Pos&Neg seq extract in subsystem 1/1(RizPos) -> Scope5/1, [IpPos]
  Igt/1 -> [Igtabc]
  [Vriz] -> "Pos&Neg seq extract in subsystem "/1(RIZ)
  [freq] -> "Pos&Neg seq extract in subsystem "/2(ffc)
  [IpRIZ] -> Pos&Neg seq extract in subsystem 1/1(RIZ)
  [freq] -> Pos&Neg seq extract in subsystem 1/2(ffc)
  [Igtabc] -> ABC_To_RIZ2/1(ABC)
  ABC_To_RIZ2/1(RIZ) -> [IgtRIZ]
  [IgtRIZ] -> Pos&Neg seq extract in subsystem 2/1(RIZ)
  [freq] -> Pos&Neg seq extract in subsystem 2/2(ffc)
  From34/1 -> Zero seq compensation/1(IgRIZ)
  From27/1 -> Pos Compensation/3(IpPos)
  From25/1 -> Pos Compensation/2(IgPos)
  From7/1 -> Pos Compensation/1(VpPos)
  Zero seq compensation/1(IpZrRef) -> Goto5/1
  Neg seq compensation/2(IpImNegRef) -> Scope1/2, Goto11/1
  Pos Compensation/1(IpRePosRef) -> Scope6/1, Goto7/1
  From29/1 -> Zero seq compensation/2(IpRIZ)
  Pos Compensation/2(IpImPosRef) -> Scope6/2, Goto8/1
  From24/1 -> Zero seq compensation/3(IrizLmtPU)
  From28/1 -> Neg seq compensation/2(IpNeg)
  Neg seq compensation/1(IpReNegRef) -> Scope1/1, Goto10/1
  Vdcs/1 -> [Vdc]
  [VdcLP] -> Subsystem5/2(Vdc)
  [Vdc] -> Scope2/3
  From37/1 -> Pos Compensation/4(Vdc)
  From38/1 -> Neg seq compensation/3(wt)
  From41/1 -> Zero seq compensation/4(Freq)
  Add/1 -> [IpReRef]
  Add1/1 -> [IpImRef]
  [IpReRef] -> Mux2/1
  Mux2/1 -> Gain2/1
  Gain2/1 -> [IpRefPU]
  [Ipabc] -> Gain3/1
  Gain3/1 -> [IpabcPU]
  [IpRIZ] -> Gain4/1
  Gain4/1 -> [IprizPU]
  [Vriz] -> Gain5/1
  Gain5/1 -> [VrizPU]
  From26/1 -> Neg seq compensation/1(IgNeg)
  [IpImRef] -> Mux2/2
  From31/1 -> PR CSI Loop/3(IrizDrp)
  [IpImPosRef] -> Add1/1
  [IpRePosRef] -> Add/1
  From30/1 -> Pos Compensation/5(wt)
  VdcsLP/1 -> [VdcLP]
  "Freq "/1 -> Scope4/1, [freq]
  wt/1 -> Scope4/2, [wt]
  VdPosPU/1 -> Gain6/1
  Gain6/1 -> [VdPosPLL]
  [Vdc] -> Pos Compensation1/1(Vdc)
  [wt] -> Pos Compensation1/2(wt)
  Pos Compensation1/1(VabcFBPU) -> [VabcFBPU]
  [VabcBPFPU] -> Sum/2
  [IpPos] -> DQ0_To_RIZ/1(DQ0)
  [wt] -> DQ0_To_RIZ/2(wt)
  DQ0_To_RIZ/1(RIZ) -> Scope/1
  [IpRIZ] -> Pos Compensation1/3(Ipriz)
  VrizBPFPU/1 -> [VrizBPFPU]

== system CSI_0313_SDC/AIP1/Subsystem5/PLL ==
  Vabc : Inport
  ABC_To_RIZ : MATLAB Function  TreatAsAtomicUnit=on
  Constant : Constant  Value=2*pi*fFqBase  SampleTime=-1
  Constant1 : Constant  Value=2*pi
  Delay1 : Delay  DelayLength=1
  Delay2 : Delay  DelayLength=1
  Demux3 : Demux  Outputs=3
  Gain : Gain  Gain=1/(2*pi)
  Integral : MATLAB Function  TreatAsAtomicUnit=on  mask{fGain=1.0, fTs=fTs}
      mask prompts: fGain "Gain Value"; fTs "Sampling time [s]"
      mask help: Proportional Resonant Controller
  Math Function : Math  Operator=mod  SaturateOnIntegerOverflow=on
  PI Ctrl : MATLAB Function  TreatAsAtomicUnit=on  mask{fKP=fKPPLL, fKI=fKIPLL, fMinLmt=fDltMin, fMaxLmt=fDltMax, fTs=fTs}
      mask prompts: fKP "Proportional Gain"; fKI "Integral Coefficient"; fMinLmt "Minimum Limitation"; fMaxLmt "Maximum Limitation"; fTs "Sampling time [s]"
      mask help: Proportional Resonant Controller
  "Pos&Neg seq extract in subsystem " : Subsystem  mask{fQ=1.0, fTs=fTs}
      mask prompts: fQ "Quality Factor"; fTs "Sample Time"
  RIZ_To_DQ0 : MATLAB Function  TreatAsAtomicUnit=on  mask{iAxis=orient 90 degree behind A-axis}
      mask prompts: iAxis "Orient Axis Choice"
  Scope : Scope
  Sum : Sum  Inputs=++|
  Terminator : Terminator
  Terminator1 : Terminator
  f : Outport
  wt : Outport  Port=2
  VdPos : Outport  Port=3
  wires:
  Delay1/1 -> "Pos&Neg seq extract in subsystem "/2(ffc)
  "Pos&Neg seq extract in subsystem "/3(chk) -> [chk]
  [f] -> Delay1/1
  Demux3/3 -> Terminator1/1
  "Pos&Neg seq extract in subsystem "/2(RizNeg) -> Terminator/1
  "Pos&Neg seq extract in subsystem "/1(RizPos) -> VdPos/1, [VrizPos]
  [Vriz] -> "Pos&Neg seq extract in subsystem "/1(RIZ)
  RIZ_To_DQ0/1(DQ0) -> Scope/1, [Vdq0Pos]
  [w] -> Gain/1
  [w] -> Integral/1(u)
  Gain/1 -> [f]
  Demux3/2 -> [VqPos]
  Demux3/1 -> [VdPos]
  [Vdq0Pos] -> Demux3/1
  PI Ctrl/1(y) -> Sum/2
  Sum/1 -> [w]
  [VrizPos] -> RIZ_To_DQ0/1(RIZ)
  Constant/1 -> Sum/1
  Vabc/1 -> [Vabc]
  Integral/1(y) -> Math Function/1
  Constant1/1 -> Math Function/2
  Math Function/1 -> [wt]
  [VqPos] -> PI Ctrl/1(err)
  [f] -> f/1
  [wt] -> Delay2/1
  Delay2/1 -> RIZ_To_DQ0/2(wt)
  [Vabc] -> ABC_To_RIZ/1(ABC)
  ABC_To_RIZ/1(RIZ) -> [Vriz]
  [wt] -> wt/1
